simulink model "problem4"  (R2020b)
settings: Solver=VariableStepAuto  StartTime=0.0  StopTime=10.0  RelTol=1e-3
libraries: simulink x2
settings Model: Creator=Administrator  LastModifiedBy=Administrator

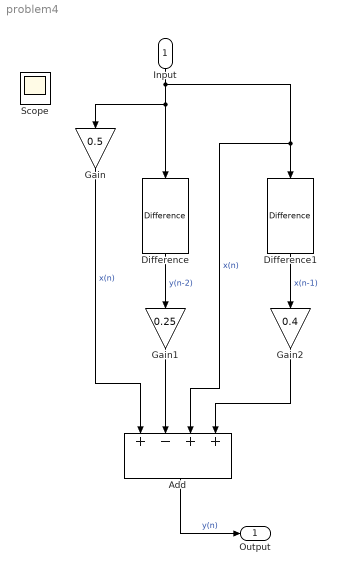
== system problem4 ==
  Input : Inport
  Add : Sum  Inputs=+-++
  Difference : simulink/Discrete/Difference  ICPrevInput=5  OutMin=[]  OutMax=[]  OutDataType=fixdt(1, 16)  OutScaling=2^-10  DoSatur=off
  Difference1 : simulink/Discrete/Difference  ICPrevInput=1  OutMin=[]  OutMax=[]  OutDataType=fixdt(1, 16)  OutScaling=2^-10  DoSatur=off
  Gain : Gain  Gain=0.5
  Gain1 : Gain  Gain=0.25
  Gain2 : Gain  Gain=0.4
  Output : Outport
  Scope : Scope
  wires:
  Difference1/1 -> Gain2/1  "x(n-1)"
  Difference/1 -> Gain1/1  "y(n-2)"
  Gain/1 -> Add/1  "x(n)"
  Gain1/1 -> Add/2
  Gain2/1 -> Add/4
  Input/1 -> Add/3, Difference1/1, Gain/1, Difference/1  "x(n)"
  Add/1 -> Output/1  "y(n)"
